simulink library "NullAircraftStateBus"  (R2018b)
settings: Solver=VariableStepAuto  StartTime=0.0  StopTime=10.0  RelTol=1e-3
libraries: signalsLib x1
settings Model: Creator=RA24876  LastModifiedBy=RA24876
settings SFSimCC: SimUseLocalCustomCode=off
settings RTWCC: RTWUseLocalCustomCode=off
settings CodeAppCC: StateflowObjectComments=on

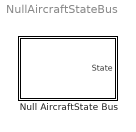
== system NullAircraftStateBus ==
  Null AircraftState Bus : Subsystem  mask(Null AircraftState Bus){}
      mask help: Creates an AircraftState bus signal with all null values. Assign values to elements with a Bus Assignment block.

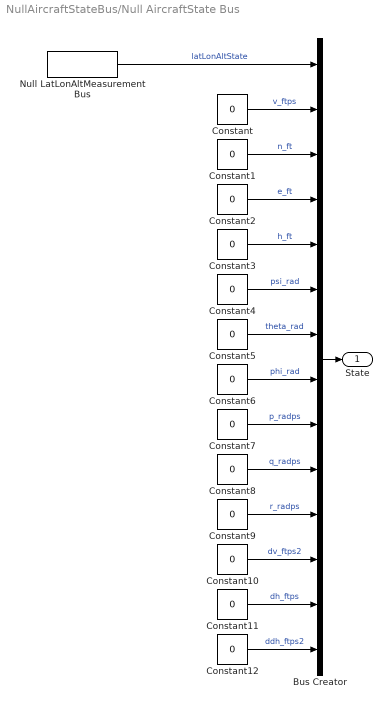
== system NullAircraftStateBus/Null AircraftState Bus ==
  Bus Creator : BusCreator  Inputs='latLonAltState','v_ftps','n_ft','e_ft','h_ft','psi_rad','theta_rad','phi_rad','p_radps','q_radps','r_radps','dv_ftps2','dh_ftps','ddh_ftps2'  OutDataTypeStr=Bus: AircraftState
  Constant{,1..12} (13 alike) : Constant  Value=0
  Null LatLonAltMeasurement Bus : signalsLib/Signals/Bus Constructors/Null LatLonAltMeasurement Bus
      settings: SourceProductName=CASSATTv6: Signals Library
  State : Outport  OutDataTypeStr=Bus: AircraftState
  wires:
  Null LatLonAltMeasurement Bus/1 -> Bus Creator/1  "latLonAltState"
  Constant/1 -> Bus Creator/2  "v_ftps"
  Constant12/1 -> Bus Creator/14  "ddh_ftps2"
  Constant1/1 -> Bus Creator/3  "n_ft"
  Bus Creator/1 -> State/1
  Constant6/1 -> Bus Creator/8  "phi_rad"
  Constant10/1 -> Bus Creator/12  "dv_ftps2"
  Constant7/1 -> Bus Creator/9  "p_radps"
  Constant5/1 -> Bus Creator/7  "theta_rad"
  Constant4/1 -> Bus Creator/6  "psi_rad"
  Constant8/1 -> Bus Creator/10  "q_radps"
  Constant9/1 -> Bus Creator/11  "r_radps"
  Constant3/1 -> Bus Creator/5  "h_ft"
  Constant2/1 -> Bus Creator/4  "e_ft"
  Constant11/1 -> Bus Creator/13  "dh_ftps"
